simulink model "singlePhasePLL"  (R2021b)
settings: Solver=ode23tb  StartTime=0  StopTime=2  FixedStep=5e-7  RelTol=1e-3  EnableMultiTasking=on
undefined symbols (not defined in the file or in its folder): sigbuilder_block
settings Model: ModifiedByFormat=Aravindh Vishnu  ModifiedComment=SESIAYY -- Tue Feb 01 14:46:59 2022 -- Version 7.0  Creator=Aravindh Vishnu  LastModifiedBy=Aravindh Vishnu
settings Model: ModifiedHistory=|
  | searvis -- Mon Jan 14 10:48:28 2019 -- Version 1.6702
  | 
  | searvis -- Mon Jan 14 10:29:06 2019 -- Version 1.6701
  | 
  | searvis -- Mon Jan 14 10:27:28 2019 -- Version 1.6700
  | 
  | searvis -- Mon Jan 14 10:26:10 2019 -- Version 1.6698
  | 
  | searvis -- Mon Jan 14 10:26:10 2019 -- Version 1.6698
  | 
  | searvis -- Mon Jan 14 10:25:48 2019 -- Version 1.6697
  | 
  | searvis -- Sat Dec 22 21:19:32 2018 -- Version 1.6696
  | 
  | searvis -- Sat Dec 22 21:19:07 2018 -- Version 1.6695
settings SolverCC: AlgebraicLoopSolver=TrustRegion
settings DataIOCC: FinalStateName=state_p3  InitialState=state_p3  SaveFormat=Array  SignalLoggingSaveFormat=ModelDataLogs  SaveOutput=off  SignalLogging=off  SaveTime=off  ReturnWorkspaceOutputs=off  SignalLoggingName=sigsOut
settings OptimizationCC: BlockReduction=off  DefaultParameterBehavior=Inlined  InlineInvariantSignals=on  BufferReuse=off  ExpressionDepthLimit=2147483647  InitFltsAndDblsToZero=on  LifeSpan=inf
settings DebuggingCC: SaveWithParameterizedLinksMsg=none  UnderspecifiedInitializationDetection=Classic  MergeDetectMultiDrivingBlocksExec=none  SignalResolutionControl=TryResolveAllWithWarning  MultiTaskDSMMsg=warning  MultiTaskCondExecSysMsg=none  FcnCallInpInsideContextMsg=warning  StateNameClashWarn=warning  SFUnexpectedBacktrackingDiag=warning  SFNoUnconditionalDefaultTransitionDiag=warning  SFExecutionAtInitializationDiag=none  SFMachineParentedDataDiag=warning  ArithmeticOperatorsInVariantConditions=warning
settings HardwareCC: ProdBitPerPointer=32  ProdBitPerSizeT=32  ProdBitPerPtrDiffT=32  ProdLargestAtomicFloat=None  ProdIntDivRoundTo=Undefined  ProdEndianess=Unspecified  ProdWordSize=32  ProdHWDeviceType=Generic->32-bit Real-Time Simulator  TargetBitPerPointer=64  TargetBitPerSizeT=64  TargetBitPerPtrDiffT=64  TargetLongLongMode=on  TargetIntDivRoundTo=Zero  TargetEndianess=LittleEndian  TargetWordSize=64  TargetHWDeviceType=MATLAB Host  ProdEqTarget=off
settings ModelReferenceCC: PropagateSignalLabelsOutOfModel=off
settings SFSimCC: SimUseLocalCustomCode=off  SimParseCustomCode=off  CustomCodeUndefinedFunction=UseInterfaceOnly
settings RTWCC: RTWUseLocalCustomCode=off
settings CodeAppCC: StateflowObjectComments=on
settings GRTTargetCC: TargetFcnLib=ansi_tfl_tmw.mat  TargetLangStandard=C89/C90 (ANSI)  CombineOutputUpdateFcns=off  GRTInterface=on
settings ConfigComp: CovMetricSettings=dw  CovSaveCumulativeToWorkspaceVar=on  CovSaveSingleToWorkspaceVar=on  CovExternalEMLEnable=off
settings SimscapeCC: SimscapeNormalizeSystem=off

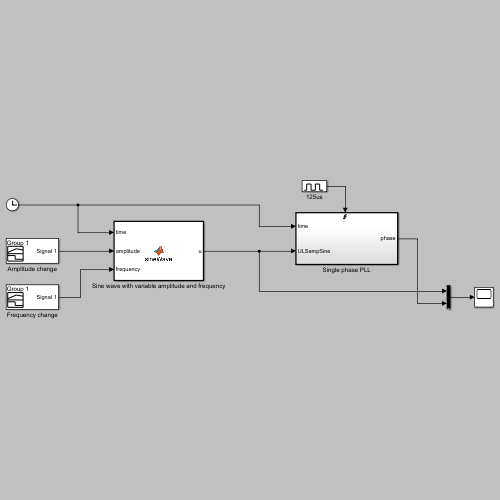
[thumbnail: Simulink's stored preview of the top-level diagram]
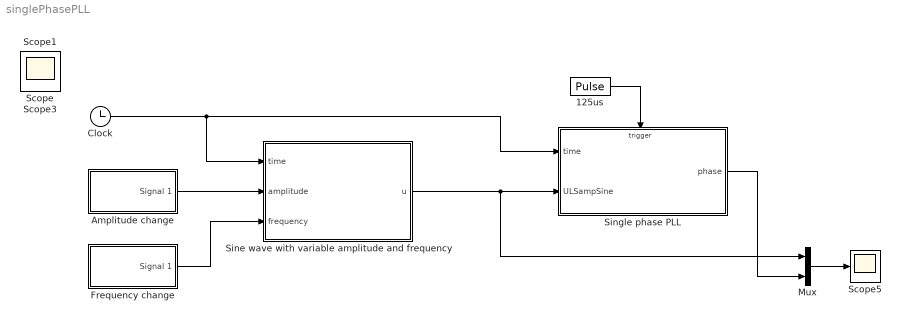
== system singlePhasePLL ==
  125us : DiscretePulseGenerator  PulseType=Time based  Period=125e-6  PulseWidth=50
  Amplitude change : Subsystem  Tag=STV Subsys  LoadFcn=sigbuilder_block('load');  StartFcn=sigbuilder_block('start');  StopFcn=sigbuilder_block('stop');  ClipboardFcn=sigbuilder_block('clipboard');  mask(Sigbuilder block){tuvar=[0:10]}
      mask help: Simulink:masks:SigbuilderBlock_MD
      mask init:
      | if ~strcmp(get_param(bdroot(gcbh),'SimulationStatus'),'stopped') tuvar = sigbuilder_block('maskInit'); end
      settings: CopyFcn=sigbuilder_block('copy');  DeleteFcn=sigbuilder_block('delete');  ModelCloseFcn=sigbuilder_block('modelClose');  PreSaveFcn=sigbuilder_block('preSave');  PauseFcn=sigbuilder_block('pause');  ContinueFcn=sigbuilder_block('continue');  NameChangeFcn=sigbuilder_block('namechange');  OpenFcn=sigbuilder_block('open',[437.6 199.2 550.4 400 ]);  CloseFcn=sigbuilder_block('close');
      mask Display: plot(0, 0, 100, 100,[2, 2, 32, 32, 2], [68, 8, 8, 68, 68],[32, 2], [38, 38], [32, 19, 2],[53, 60, 44], [32, 17, 17, 2],[16, 16, 31, 31]);txt = getActiveGroup(gcbh);text(2, 100, txt,'verticalAlignment', 'top');
  Clock : Clock
  Frequency change : Subsystem  Tag=STV Subsys  LoadFcn=sigbuilder_block('load');  StartFcn=sigbuilder_block('start');  StopFcn=sigbuilder_block('stop');  ClipboardFcn=sigbuilder_block('clipboard');  mask(Sigbuilder block){tuvar=[0:10]}
      mask help: Simulink:masks:SigbuilderBlock_MD
      mask init:
      | if ~strcmp(get_param(bdroot(gcbh),'SimulationStatus'),'stopped') tuvar = sigbuilder_block('maskInit'); end
      settings: CopyFcn=sigbuilder_block('copy');  DeleteFcn=sigbuilder_block('delete');  ModelCloseFcn=sigbuilder_block('modelClose');  PreSaveFcn=sigbuilder_block('preSave');  PauseFcn=sigbuilder_block('pause');  ContinueFcn=sigbuilder_block('continue');  NameChangeFcn=sigbuilder_block('namechange');  OpenFcn=sigbuilder_block('open',[437.6 199.2 550.4 400 ]);  CloseFcn=sigbuilder_block('close');
      mask Display: plot(0, 0, 100, 100,[2, 2, 32, 32, 2], [68, 8, 8, 68, 68],[32, 2], [38, 38], [32, 19, 2],[53, 60, 44], [32, 17, 17, 2],[16, 16, 31, 31]);txt = getActiveGroup(gcbh);text(2, 100, txt,'verticalAlignment', 'top');
  Mux : Mux  Inputs=2
  Scope{,1,3,5} (4 alike) : Scope
  Sine wave with variable amplitude and frequency : MATLAB Function  TreatAsAtomicUnit=on
  Single phase PLL : Subsystem
  wires:
  125us/1 -> Single phase PLL/Trigger
  Single phase PLL/1(phase) -> Mux/2
  Mux/1 -> Scope5/1
  Frequency change/1(Signal 1) -> Sine wave with variable amplitude and frequency/3(frequency)
  Sine wave with variable amplitude and frequency/1(u) -> Mux/1, Single phase PLL/2(ULSampSine)
  Clock/1 -> Sine wave with variable amplitude and frequency/1(time), Single phase PLL/1(time)
  Amplitude change/1(Signal 1) -> Sine wave with variable amplitude and frequency/2(amplitude)

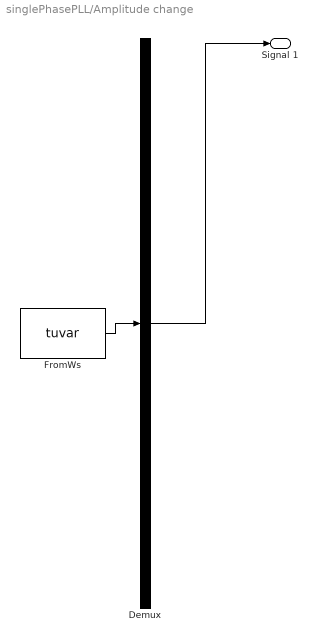
== system singlePhasePLL/Amplitude change ==
  Demux : Demux  Tag=STV Demux  Outputs=1
      settings: DisplayOption=none
  FromWs : FromWorkspace  Tag=STV FromWs  VariableName=tuvar
      SigBuilderData=|
      | common.afterFinalStr = 'Extrapolate'
      | common.sampleTime = 0
      | dataSet.timeRange = [0 2]
      | dataSet.name = 'Group 1'
      | sbobj.Groups.Name = 'Group 1'
      | sbobj.Groups.Signals.Name = 'Signal 1'
      | sbobj.Groups.Signals.XData = [0 1 2]
      | sbobj.Groups.Signals.YData = [1 2 1]
      | sbobj.Groups.TimeRange = [0 2]
  Signal 1 : Outport  Tag=STV Outport  VectorParamsAs1DForOutWhenUnconnected=off
  wires:
  Demux/1 -> Signal 1/1
  FromWs/1 -> Demux/1

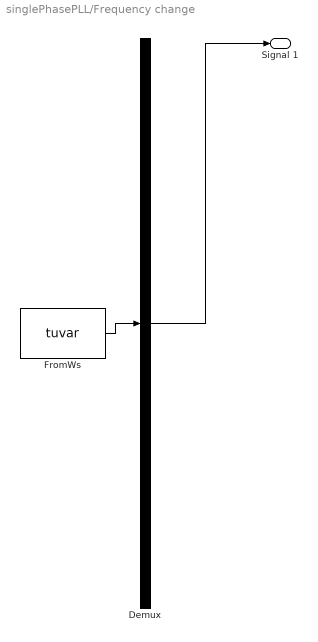
== system singlePhasePLL/Frequency change ==
  Demux : Demux  Tag=STV Demux  Outputs=1
      settings: DisplayOption=none
  FromWs : FromWorkspace  Tag=STV FromWs  VariableName=tuvar
      SigBuilderData=|
      | common.afterFinalStr = 'Extrapolate'
      | common.sampleTime = 0
      | dataSet.timeRange = [0 2]
      | dataSet.name = 'Group 1'
      | sbobj.Groups.Name = 'Group 1'
      | sbobj.Groups.Signals.Name = 'Signal 1'
      | sbobj.Groups.Signals.XData = [0 0.5 1.5 2]
      | sbobj.Groups.Signals.YData = [55 50 60 55]
      | sbobj.Groups.TimeRange = [0 2]
  Signal 1 : Outport  Tag=STV Outport  VectorParamsAs1DForOutWhenUnconnected=off
  wires:
  Demux/1 -> Signal 1/1
  FromWs/1 -> Demux/1

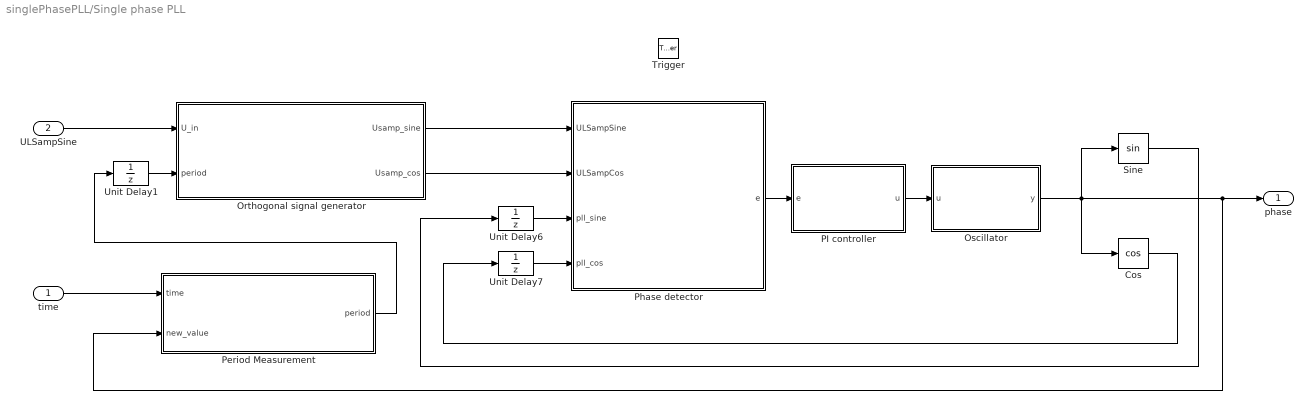
== system singlePhasePLL/Single phase PLL ==
  time : Inport
  ULSampSine : Inport  Port=2
  Trigger : TriggerPort  VariantControl=Variant
  Cos : Trigonometry  Operator=cos
  Orthogonal signal generator : MATLAB Function  TreatAsAtomicUnit=on
  Oscillator : MATLAB Function  TreatAsAtomicUnit=on
  PI controller : Subsystem
  Period Measurement : MATLAB Function  TreatAsAtomicUnit=on
  Phase detector : MATLAB Function  TreatAsAtomicUnit=on
  Sine : Trigonometry
  Unit Delay1 : UnitDelay  SampleTime=-1  HasFrameUpgradeWarning=on
  Unit Delay6 : UnitDelay  SampleTime=-1  HasFrameUpgradeWarning=on
  Unit Delay7 : UnitDelay  SampleTime=-1  HasFrameUpgradeWarning=on
  phase : Outport  VectorParamsAs1DForOutWhenUnconnected=off
  wires:
  Oscillator/1(y) -> phase/1, Period Measurement/2(new_value), Sine/1, Cos/1
  Sine/1 -> Unit Delay6/1
  Cos/1 -> Unit Delay7/1
  Unit Delay6/1 -> Phase detector/3(pll_sine)
  Unit Delay7/1 -> Phase detector/4(pll_cos)
  time/1 -> Period Measurement/1(time)
  ULSampSine/1 -> Orthogonal signal generator/1(U_in)
  Orthogonal signal generator/2(Usamp_cos) -> Phase detector/2(ULSampCos)
  Orthogonal signal generator/1(Usamp_sine) -> Phase detector/1(ULSampSine)
  Unit Delay1/1 -> Orthogonal signal generator/2(period)
  Period Measurement/1(period) -> Unit Delay1/1
  Phase detector/1(e) -> PI controller/1(e)
  PI controller/1(u) -> Oscillator/1(u)

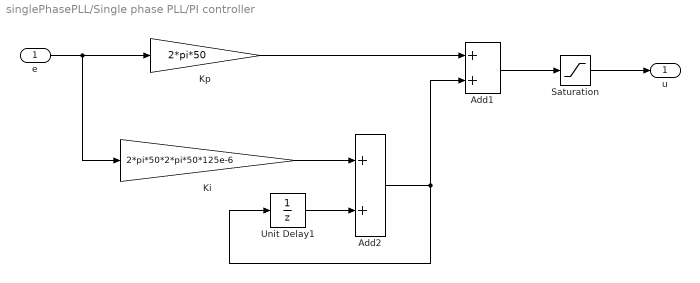
== system singlePhasePLL/Single phase PLL/PI controller ==
  e : Inport
  Add1 : Sum
  Add2 : Sum
  Ki : Gain  Gain=2*pi*50*2*pi*50*125e-6
  Kp : Gain  Gain=2*pi*50
  Saturation : Saturate  UpperLimit=1100  LowerLimit=-1100
  Unit Delay1 : UnitDelay  SampleTime=-1  HasFrameUpgradeWarning=on
  u : Outport  VectorParamsAs1DForOutWhenUnconnected=off
  wires:
  Saturation/1 -> u/1
  Kp/1 -> Add1/1
  Add1/1 -> Saturation/1
  Add2/1 -> Unit Delay1/1, Add1/2
  Ki/1 -> Add2/1
  Unit Delay1/1 -> Add2/2
  e/1 -> Ki/1, Kp/1

== matlab function singlePhasePLL/Single phase PLL/Phase detector ==
  data: e output; ULSampSine input; ULSampCos input; pll_sine input; pll_cos input
function e  = phaseDetector(ULSampSine, ULSampCos, pll_sine, pll_cos)

r = ULSampSine * pll_cos;
y = ULSampCos * pll_sine;
e = r -y;

end

== matlab function singlePhasePLL/Single phase PLL/Period Measurement ==
  data: time input; new_value input; period output size=1
function period = periodMeasurement(time,new_value)
% Period measurement

% The persistent variables are retained in memory before calls to the function
persistent previous_value;
persistent previous_zerocross;
persistent new_zerocross;
persistent period_fp;
persistent previous_time

% Initialize the persistent variables
if isempty(previous_value)
    previous_value = 0;
    previous_zerocross = 0;
    new_zerocross = 0;
    period_fp = 0.018;
    previous_time = 0;
end

new_value = new_value - pi;

if (new_value < 0 && previous_value >= 0)
        
    t_1 = time;

    t_2 = previous_time;

    new_zerocross = ((((0 - previous_value) * (t_1 - t_2))/(new_value - previous_value)) + t_2);

    period_fp = new_zerocross - previous_zerocross;
        
end

period = period_fp;

previous_zerocross = new_zerocross;

previous_value = new_value;

previous_time = time;

end

== matlab function singlePhasePLL/Single phase PLL/Oscillator ==
  data: u input; y output
function y = oscillator(u)

persistent previous_value;

DELTA = 125e-6;

if isempty(previous_value)
    previous_value = 0;
end

current_value = u * DELTA + previous_value;
y = mod(current_value,2*pi);

previous_value = current_value;

end

== matlab function singlePhasePLL/Sine wave with variable amplitude and frequency ==
  data: time input; amplitude input; frequency input; u output size=1
function u = sineWave(time,amplitude,frequency)

% Sine waveform with variable frequency and amplitude
u = amplitude * sin(2 * pi * frequency * time);

end

== matlab function singlePhasePLL/Single phase PLL/Orthogonal signal generator ==
  data: Usamp_sine output; U_in input; period input; Usamp_cos output
function [Usamp_sine, Usamp_cos] = orthogonalSignalGenerator(U_in, period)

BUFFER_SIZE = 300;
SAMPLE_TIME = 125e-6;

% The persistent variables are retained in memory before calls to the function
persistent array_values_U;
persistent voltage_meas_last_index;

% Initialize the persistent variables
if isempty(voltage_meas_last_index)
    array_values_U = zeros(BUFFER_SIZE, 1);
    voltage_meas_last_index = 0;
end

% Execute the buffer and start storing the data
voltage_meas_last_index = voltage_meas_last_index + 1;
if (voltage_meas_last_index == BUFFER_SIZE+1)
    voltage_meas_last_index = 1;
end

array_values_U(voltage_meas_last_index) = U_in;

Usamp_sine = array_values_U(voltage_meas_last_index);

% Number of samples per period
num_of_samples = period / SAMPLE_TIME;

degree_back_90 = round(num_of_samples / 4);

if (voltage_meas_last_index - degree_back_90 <= 1)
    index_90 = (BUFFER_SIZE - (degree_back_90 - voltage_meas_last_index) - 1);
else
	index_90 = voltage_meas_last_index - degree_back_90 - 1;
end

Usamp_cos = array_values_U(index_90);
Usamp_cos = -Usamp_cos;

end
